simulink model "verify_StorageTnodesEN12977losses_mdl"  (R2018b)
settings: Solver=ode45  StartTime=0.0  StopTime=400*3600  MaxStep=60  RelTol=1e-3  EnableMultiTasking=on
libraries: carnot x3
settings Model: Creator=drhf  LastModifiedBy=drhf
settings DataIOCC: SaveFormat=Array  SignalLoggingSaveFormat=ModelDataLogs
settings OptimizationCC: ExpressionDepthLimit=2147483647  LifeSpan=inf
settings DebuggingCC: UnderspecifiedInitializationDetection=Classic  MergeDetectMultiDrivingBlocksExec=none  SolverPrmCheckMsg=warning  FcnCallInpInsideContextMsg=warning  StateNameClashWarn=warning  SFUnexpectedBacktrackingDiag=warning  SFNoUnconditionalDefaultTransitionDiag=warning  SFExecutionAtInitializationDiag=none
settings HardwareCC: ProdBitPerPointer=32  ProdBitPerSizeT=32  ProdBitPerPtrDiffT=32  ProdLargestAtomicFloat=None  ProdIntDivRoundTo=Undefined  ProdEndianess=Unspecified  ProdWordSize=32  ProdHWDeviceType=32-bit Generic
settings ModelReferenceCC: PropagateSignalLabelsOutOfModel=off
settings SFSimCC: SimUseLocalCustomCode=off
settings RTWCC: RTWUseLocalCustomCode=off
settings CodeAppCC: StateflowObjectComments=on
settings GRTTargetCC: TargetLangStandard=C89/C90 (ANSI)  GeneratePreprocessorConditionals=Disable all  CombineOutputUpdateFcns=off  GRTInterface=on
settings ConfigComp: CovMetricSettings=dw  CovHtmlReporting=on  CovSaveCumulativeToWorkspaceVar=on  CovSaveSingleToWorkspaceVar=on  CovExternalEMLEnable=off

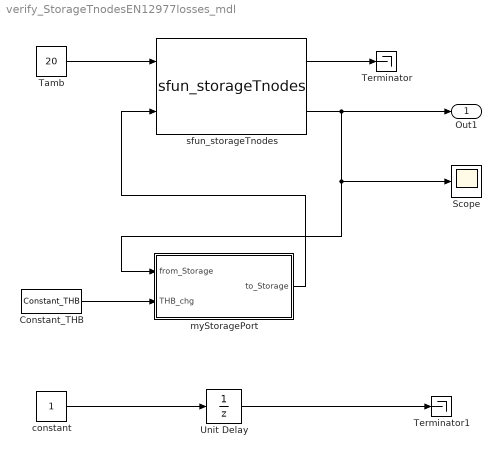
== system verify_StorageTnodesEN12977losses_mdl ==
  Constant_THB : carnot/Source/Simple/Constant_THB  t=40  mdot=0  p=1e5  mID=No Pressure Drop  fluid=Water (Constant 20°C)  mix=0  mix2=0  mix3=0  dia=0.02  hgt=0
      settings: SourceProductName=Carnot
  Scope : Scope
  Tamb : Constant  Value=20
  Terminator : Terminator
  Terminator1 : Terminator
  Unit Delay : UnitDelay  SampleTime=3600
  constant : Constant
  myStoragePort : Subsystem  mask(Multiport Storage){uloss=1, ubot=1, utop=1, cond=1, t0=20, volume=0.3, dia=0.5, pos=standing cylinder, nconnect=1, nodes=1, mpoints=1}
      mask prompts: uloss "Heat loss coefficient cylinder wall in W/(m²K)"; ubot "Heat loss coefficient bottom in W/(m²K)"; utop "Heat loss coefficient top cover in W/(m²K)"; cond "Effective vertical conductivity in W/(m*K)"; t0 "Initial temperature (vector or scalar) in °C"; volume "Volume in m³"; dia "Diameter in m"; pos "Position"; nconnect "Number of connections"; nodes "Number of nodes"; mpoints "Number of measurement points"
      mask help:
      | The volmue of the cylindrical storage is divided in a number "nodes" of horizontal slices (1xN-node model). For each node the energy balance equation is solved.
      | Look under mask to set the ports types and properties.
      mask init:
      | % [standing, dh, height, mpts, tini] ...
      | %     = CarnotCallbacks_StorageTypeN(pos, volume, dia, nodes, mpoints, t0);
      | standing = pos-1;
      | if standing
      |     dh = volume/(0.25*dia^2*pi*nodes);
      | else
      |     dh = dia/nodes;
      | end
      | height = dh*nodes;
      | mpoints = max(mpoints,1);
      | mpts = round(nodes/mpoints/2:nodes/mpoints:nodes);
      | n0 = length(t0);
      | if n0 > 1
      |     x = linspace(0,1,n0);
      |     xx = linspace(0,1,nodes);
      |     tini = spline(x,t0,xx);
      |     tmin = min(t0);
      |     tmax = max(t0);
      |     tini = min(tini, tmax);
      |     tini = max(tini, tmin);
      | else
      |     tini = ones(1,nodes).*t0;
      | end
      mask Help: eval('man(''storage_multiport'')')
      mask TypeOptions pos: lying cylinder | standing cylinder
      mask DialogControl ParameterTabVar0 Prompt: Thermal
      mask DialogControl ParameterTabVar01 Prompt: Geometry
      mask DialogControl ParameterTabVar012 Prompt: Calculation
  sfun_storageTnodes : carnot/Basic/Thermal_Models/sfun_storageTnodes  uloss=7  ubot=0  utop=0  cond=0  volume=0.47921  dia=0.6  standing=standing cylinder  tini=60  nodes=1  nconnect=1  elimthermocline=1  condinvtc=1e5
      settings: SourceProductName=Carnot
  Out1 : Outport
  wires:
  Tamb/1 -> sfun_storageTnodes/1
  myStoragePort/1(to_Storage) -> sfun_storageTnodes/2
  sfun_storageTnodes/2 -> Scope/1, myStoragePort/1(from_Storage), Out1/1
  Constant_THB/1 -> myStoragePort/2(THB_chg)
  sfun_storageTnodes/1 -> Terminator/1
  constant/1 -> Unit Delay/1
  Unit Delay/1 -> Terminator1/1

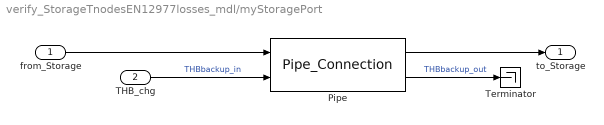
== system verify_StorageTnodesEN12977losses_mdl/myStoragePort ==
  from_Storage : Inport
  THB_chg : Inport  Port=2
  Pipe : carnot/Storage/Thermal/Storage_Ports/Pipe_Connection  h_in=1  h_out=0  hgt=height  dpipe=0.03  dstg=1  nodes=nodes
      settings: SourceProductName=Carnot
  Terminator : Terminator
  to_Storage : Outport
  wires:
  THB_chg/1 -> Pipe/2  "THBbackup_in"
  from_Storage/1 -> Pipe/1
  Pipe/1 -> to_Storage/1
  Pipe/2 -> Terminator/1  "THBbackup_out"
